simulink model "modelling"  (R2020b)
settings: Solver=ode15s  StartTime=0.0  StopTime=15  FixedStep=0.01  RelTol=1e-3
settings Model: Creator=Admin  LastModifiedBy=Admin

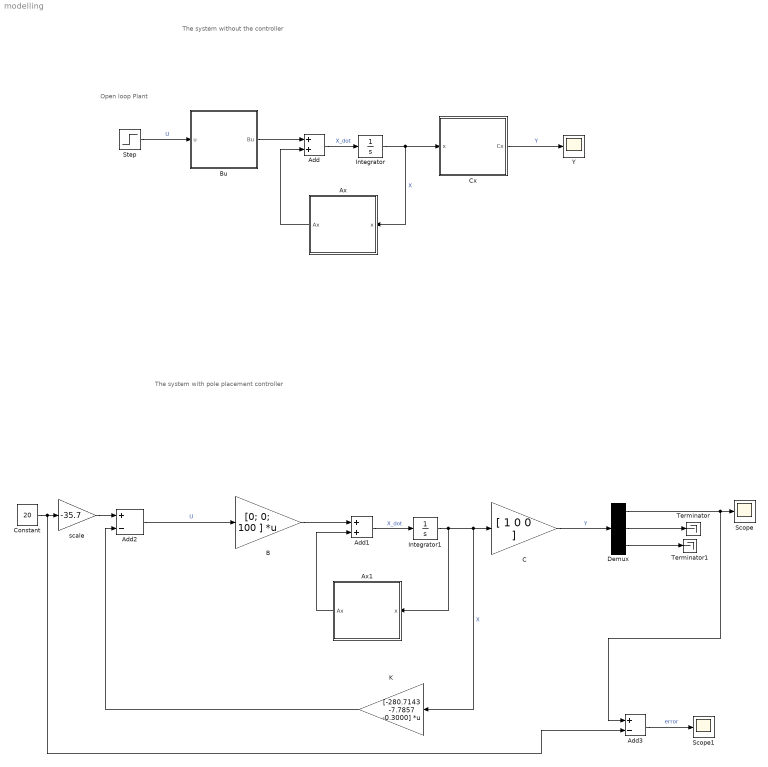
== system modelling ==
  note: Open loop Plant
  note: The system without the controller
  note: The system with pole placement controller
  Add : Sum
  Add1 : Sum
  Add2 : Sum  Inputs=+-
  Add3 : Sum  Inputs=+-
  Ax : MATLAB Function  TreatAsAtomicUnit=on
  Ax1 : MATLAB Function  TreatAsAtomicUnit=on
  B : Gain  Gain=[0; 0; 100 ]  Multiplication=Matrix(K*u)
  Bu : MATLAB Function  TreatAsAtomicUnit=on
  C : Gain  Gain=[ 1 0 0 ]
  Constant : Constant  Value=20
  Cx : MATLAB Function  TreatAsAtomicUnit=on
  Demux : Demux  Outputs=3
  Integrator : Integrator  InitialCondition=[0.01; 0; 0]
  Integrator1 : Integrator  InitialCondition=[0.1;0; 0]
  K : Gain  Gain="[-280.7143   -7.7857   -0.3000]"  Multiplication=Matrix(K*u)
  Scope : Scope
  Scope1 : Scope
  Step : Step  Time=0  After=0  SampleTime=0
  Terminator : Terminator
  Terminator1 : Terminator
  Y : Scope
  scale : Gain  Gain=-35.7
  wires:
  Integrator/1 -> Ax/1(x), Cx/1(x)  "X"
  Ax/1(Ax) -> Add/2
  Add/1 -> Integrator/1  "X_dot"
  Bu/1(Bu) -> Add/1
  Cx/1(Cx) -> Y/1  "Y"
  Step/1 -> Bu/1(u)  "U"
  B/1 -> Add1/1
  Ax1/1(Ax) -> Add1/2
  Integrator1/1 -> C/1, K/1, Ax1/1(x)  "X"
  Add1/1 -> Integrator1/1  "X_dot"
  C/1 -> Demux/1  "Y"
  Add2/1 -> B/1  "U"
  K/1 -> Add2/2
  Demux/2 -> Terminator/1
  Demux/3 -> Terminator1/1
  Constant/1 -> Add3/2, scale/1
  Demux/1 -> Add3/1, Scope/1
  scale/1 -> Add2/1
  Add3/1 -> Scope1/1  "error"

== matlab function modelling/Ax ==
  data: x input; Ax output
function Ax = fcn(x)

A  = [ 0   1   0
     980  0  -2.8
      0   0  -100 ];
  
Ax = A*x  ;

== matlab function modelling/Cx ==
  data: x input; Cx output
function Cx = fcn(x)


  
C = [ 1 0 0 ];
Cx = C*x;

== matlab function modelling/Ax1 ==
  data: x input; Ax output
function Ax = fcn(x)

A  = [ 0   1   0
     980  0  -2.8
      0   0  -100 ];
  
Ax = A*x;

== matlab function modelling/Bu ==
  data: u input; Bu output
function Bu = fcn(u)


  
B = [ 0;
      0;
      100 ];
  
Bu = B*u
